simulink model "extra_task_PID_2020"  (R2020b)
settings: Solver=FixedStepAuto  StartTime=0.0  StopTime=2000  FixedStep=0.001  RelTol=1e-3
values from neighbouring files (symbols this model uses):
  hd = 1.5    [Copy_of_Lab_3_ale.m]    (also in Lab_3_ale.m)
  hi = 0    [Copy_of_Lab_3_ale.m]    (also in Lab_3_ale.m = 0.2)
  hp = 0    [Copy_of_Lab_3_ale.m]    (also in Lab_3_ale.m)
  kp = 6.32    [Copy_of_Lab_3_ale.m]    (also in Lab_3_ale.m; mass_2dof.m)
  mp = 0.16    [Copy_of_Lab_3_ale.m]    (also in Lab_3_ale.m; mass_2dof.m)
settings Model: Creator=rivaa  LastModifiedBy=rivaa
settings DebuggingCC: SFMachineParentedDataDiag=error

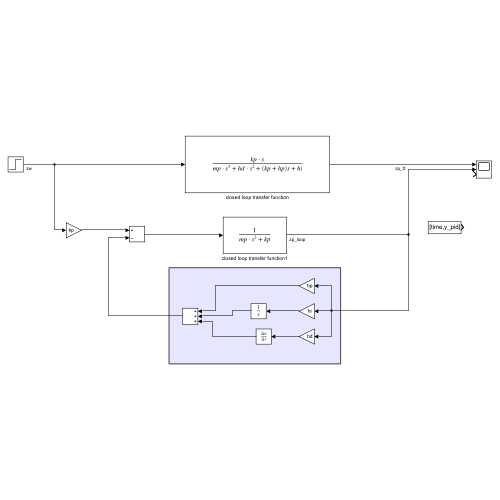
[thumbnail: Simulink's stored preview of the top-level diagram]
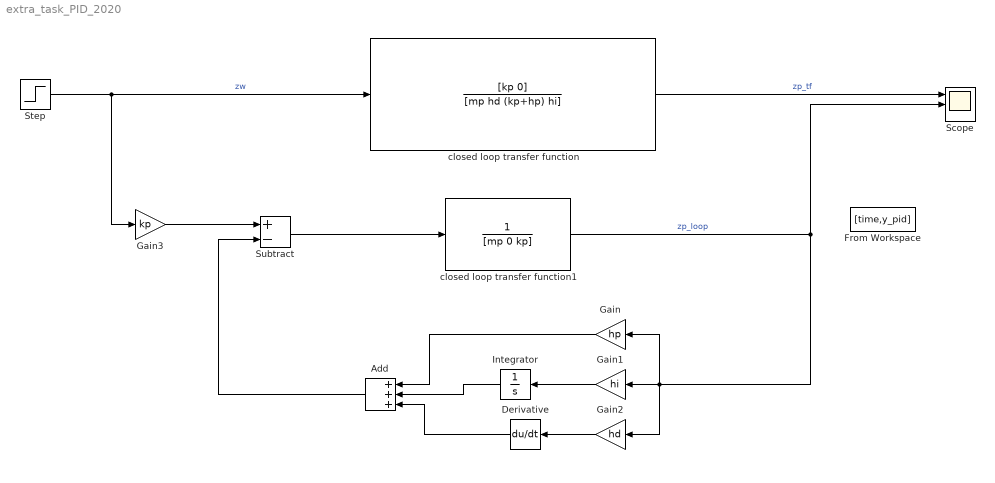
== system extra_task_PID_2020 ==
  Add : Sum  Inputs=+++
  Derivative : Derivative
  From Workspace : FromWorkspace  VariableName=[time,y_pid]
  Gain : Gain  Gain=hp
  Gain1 : Gain  Gain=hi
  Gain2 : Gain  Gain=hd
  Gain3 : Gain  Gain=kp
  Integrator : Integrator
  Scope : Scope  NumInputPorts=3
  Step : Step  Time=0  SampleTime=0
  Subtract : Sum  Inputs=+-
  closed loop transfer function : TransferFcn  Numerator=[kp 0]  Denominator=[mp hd (kp+hp) hi]
  closed loop transfer function1 : TransferFcn  Numerator=1  Denominator=[mp 0 kp]
  wires:
  Step/1 -> closed loop transfer function/1, Gain3/1  "zw"
  Gain1/1 -> Integrator/1
  Gain2/1 -> Derivative/1
  Gain/1 -> Add/1
  Integrator/1 -> Add/2
  Derivative/1 -> Add/3
  closed loop transfer function/1 -> Scope/1  "zp_tf"
  Gain3/1 -> Subtract/1
  Subtract/1 -> closed loop transfer function1/1
  closed loop transfer function1/1 -> Scope/2, Gain2/1, Gain/1, Gain1/1  "zp_loop"
  Add/1 -> Subtract/2
